simulink subsystem "theta2vector"  (R2024b)
settings: Solver=VariableStepAuto  StartTime=0.0  StopTime=10.0  RelTol=1e-3
settings Model: Creator=Asus  LastModifiedBy=Asus

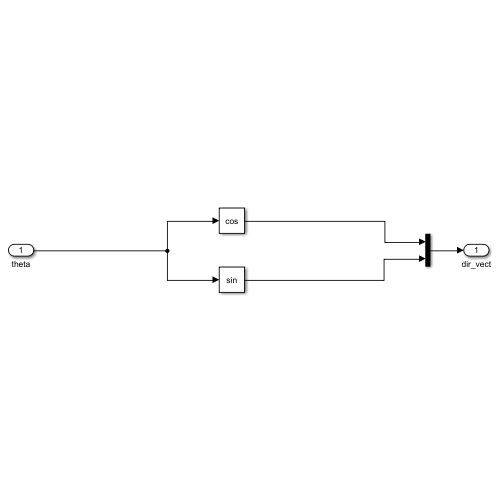
[thumbnail: Simulink's stored preview of the top-level diagram]
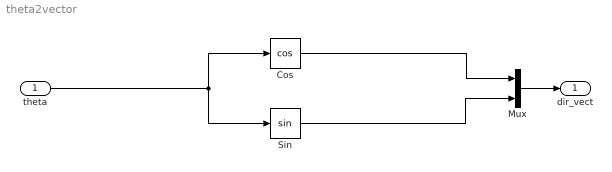
== system theta2vector ==
  theta : Inport
  Cos : Trigonometry  Operator=cos
  Mux : Mux  Inputs=2
  Sin : Trigonometry
  dir_vect : Outport
  wires:
  theta/1 -> Sin/1, Cos/1
  Mux/1 -> dir_vect/1
  Cos/1 -> Mux/1
  Sin/1 -> Mux/2
